simulink model "vtg_sim"  (R2025b)
settings: Solver=ode45  StartTime=0.0  StopTime=40.0  RelTol=1e-3
settings Model: Creator=sprinkle  LastModifiedBy=sprinkle
settings OptimizationCC: ReuseModelBlockBuffer=off
settings RTWCC: GPUComputeCapability=3.5

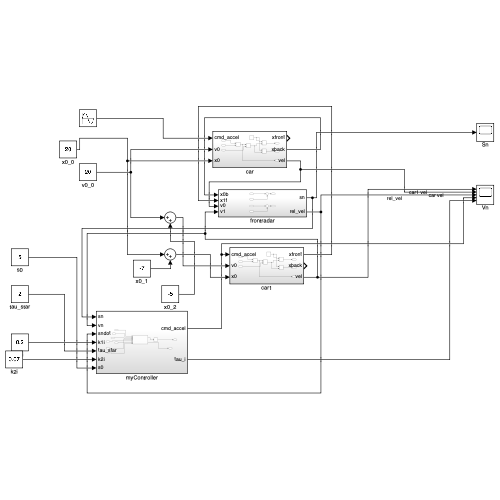
[thumbnail: Simulink's stored preview of the top-level diagram]
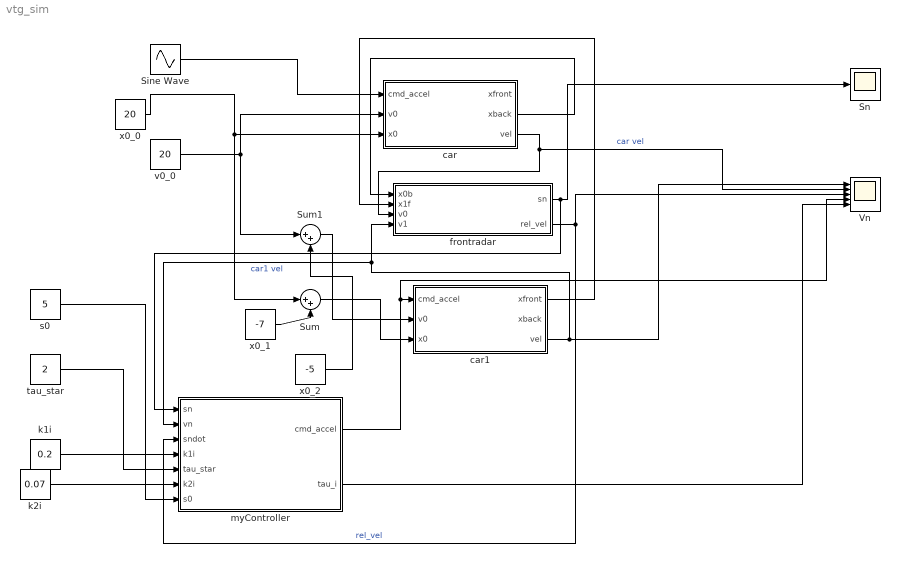
== system vtg_sim ==
  Sine Wave : Sin  Amplitude=0.25  SampleTime=0
  Sn : Scope
      settings: ActiveDisplayYMinimum=-2.6106737980670882  ActiveDisplayYMaximum=51.096064182603783
  Sum : Sum  Inputs=|++
  Sum1 : Sum  Inputs=|++
  Vn : Scope  NumInputPorts=5
      settings: ActiveDisplayYMinimum=-15.489718822251529  ActiveDisplayYMaximum=35.697668945320132
  car : Subsystem
  car1 : Subsystem
  frontradar : Subsystem
  k1i : Constant  Value=0.2
  k2i : Constant  Value=0.07
  myController : Subsystem
  s0 : Constant  Value=5
  tau_star : Constant  Value=2
  v0_0 : Constant  Value=20
  x0_0 : Constant  Value=20
  x0_1 : Constant  Value=-7
  x0_2 : Constant  Value=-5
  wires:
  Sine Wave/1 -> car/1(cmd_accel)
  v0_0/1 -> car/2(v0), Sum1/1
  x0_0/1 -> Sum/1, car/3(x0)
  x0_1/1 -> Sum/2
  Sum/1 -> car1/3(x0)
  x0_2/1 -> Sum1/2
  Sum1/1 -> car1/2(v0)
  car/2(xback) -> frontradar/1(x0b)
  car1/1(xfront) -> frontradar/2(x1f)
  car/3(vel) -> Vn/2, frontradar/3(v0)  "car vel"
  car1/3(vel) -> Vn/1, frontradar/4(v1), myController/2(vn)  "car1 vel"
  frontradar/1(sn) -> myController/1(sn), Sn/1
  frontradar/2(rel_vel) -> myController/3(sndot), Vn/3  "rel_vel"
  s0/1 -> myController/7(s0)
  tau_star/1 -> myController/5(tau_star)
  myController/1(cmd_accel) -> Vn/4, car1/1(cmd_accel)
  k1i/1 -> myController/4(k1i)
  k2i/1 -> myController/6(k2i)
  myController/2(tau_i) -> Vn/5

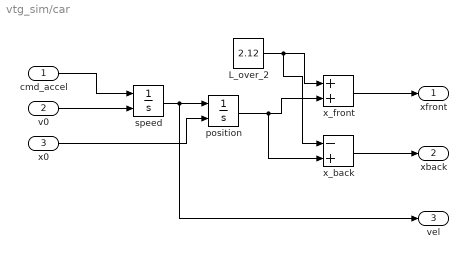
== system vtg_sim/car ==
  cmd_accel : Inport
  v0 : Inport  Port=2
  x0 : Inport  Port=3
  L_over_2 : Constant  Value=2.12
  position : Integrator  InitialConditionSource=external
  speed : Integrator  InitialConditionSource=external
  x_back : Sum  Inputs=-+
  x_front : Sum
  xfront : Outport
  xback : Outport  Port=2
  vel : Outport  Port=3
  wires:
  x_back/1 -> xback/1
  x0/1 -> position/2
  cmd_accel/1 -> speed/1
  speed/1 -> vel/1, position/1
  position/1 -> x_back/2, x_front/2
  x_front/1 -> xfront/1
  v0/1 -> speed/2
  L_over_2/1 -> x_back/1, x_front/1

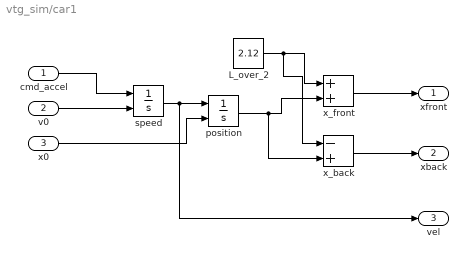
== system vtg_sim/car1 ==
  cmd_accel : Inport
  v0 : Inport  Port=2
  x0 : Inport  Port=3
  L_over_2 : Constant  Value=2.12
  position : Integrator  InitialConditionSource=external
  speed : Integrator  InitialConditionSource=external
  x_back : Sum  Inputs=-+
  x_front : Sum
  xfront : Outport
  xback : Outport  Port=2
  vel : Outport  Port=3
  wires:
  x_back/1 -> xback/1
  x0/1 -> position/2
  cmd_accel/1 -> speed/1
  speed/1 -> vel/1, position/1
  position/1 -> x_back/2, x_front/2
  x_front/1 -> xfront/1
  v0/1 -> speed/2
  L_over_2/1 -> x_back/1, x_front/1

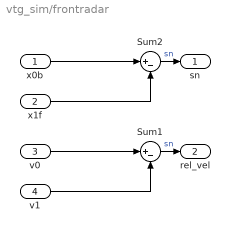
== system vtg_sim/frontradar ==
  x0b : Inport
  x1f : Inport  Port=2
  v0 : Inport  Port=3
  v1 : Inport  Port=4
  Sum1 : Sum  Inputs=|+-
  Sum2 : Sum  Inputs=|+-
  sn : Outport
  rel_vel : Outport  Port=2
  wires:
  x1f/1 -> Sum2/2
  Sum2/1 -> sn/1  "sn"
  x0b/1 -> Sum2/1
  v0/1 -> Sum1/1
  Sum1/1 -> rel_vel/1  "sn"
  v1/1 -> Sum1/2

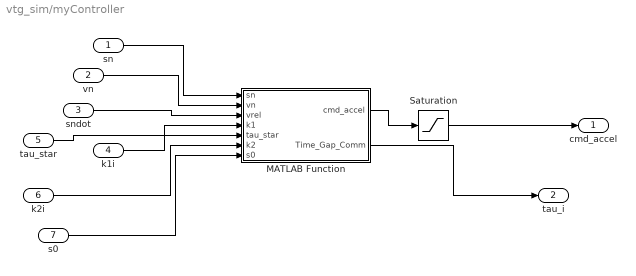
== system vtg_sim/myController ==
  sn : Inport
  vn : Inport  Port=2
  sndot : Inport  Port=3
  k1i : Inport  Port=4
  tau_star : Inport  Port=5
  k2i : Inport  Port=6
  s0 : Inport  Port=7
  MATLAB Function : MATLAB Function  TreatAsAtomicUnit=on
  Saturation : Saturate  UpperLimit=1.5  LowerLimit=-3
  cmd_accel : Outport
  tau_i : Outport  Port=2
  wires:
  MATLAB Function/1(cmd_accel) -> Saturation/1
  k1i/1 -> MATLAB Function/4(k1)
  sn/1 -> MATLAB Function/1(sn)
  vn/1 -> MATLAB Function/2(vn)
  sndot/1 -> MATLAB Function/3(vrel)
  k2i/1 -> MATLAB Function/6(k2)
  s0/1 -> MATLAB Function/7(s0)
  tau_star/1 -> MATLAB Function/5(tau_star)
  Saturation/1 -> cmd_accel/1
  MATLAB Function/2(Time_Gap_Comm) -> tau_i/1

== matlab function vtg_sim/myController/MATLAB Function ==
  data: sn input; cmd_accel output; vn input; vrel input; k1 input; tau_star input; k2 input; s0 input; Time_Gap_Comm output
function [cmd_accel, Time_Gap_Comm] = vtg_acc_fcn(sn, vn, vrel, k1, tau_star, k2, s0)

coder.extrinsic('icare'); 

rho_s = 0.2;
rho_v = 0.5;
rho_u = 1.0;
gamma = 0.95;
Asys = [0 -1; k1 (-k1*tau_star-k2)];
Bdist = [1; k2];
Csys = [rho_s 0; 0 rho_v; 0 0];
Ru = rho_u^2;
Rmat = [-1/gamma^2 0; 0 inv(Ru)];

ve = vrel + vn;
s_err = sn - (s0+tau_star*ve);
v_err = vn - ve;
Bctrl = [0; -k1*ve];
P=zeros(2);
% TODO: come up with a code-generatable ricatti equation solution
[P, ~, ~] = icare(Asys, [Bdist, Bctrl], Csys'*Csys, Rmat, [], [], []);

ui = -inv(Ru)*([0 -k1*vn]*P*[s_err; v_err]);
Time_Gap_Comm = max(tau_star + double(ui), 0);
cmd_accel = k1*(sn-s0-Time_Gap_Comm*vn) + k2*vrel;

end
